simulink model "vof_control"  (R2022b)
settings: Solver=ode4  StartTime=0.0  StopTime=20  FixedStep=0.001  RelTol=1e-3
values from neighbouring files (symbols this model uses):
  Cm = [ones(1,r),zeros(1,r)]    [modal_control.m]
  Cv1 = ci*Cv    [modal_control.m]
  f = linspace(0, Fs/2, length(datos_filt)/2+1)    [FRF.m]    (also in FRFFrequencyResponseFunction.m; fft_Acelerometro.m = Fs*(0:(L/2))/L; fft_Mocap.m = Fs*(0:(L/2))/L; fftmocap.m = Fs*(0:(L/2))/L)
  fd = 8    [modal_control.m]
  gv = -2*w(i)*zetag/(bi*ci)    [modal_control.m]
  h = 1    [modal_control.m]
  k = 2*r    (= 10)    [modal_control.m]
  wn = sqrt(diag(eigenvalues))    [PironInternet.m]
undefined symbols (not defined in the file or in its folder): Am, Bm
settings Model: Creator=Jka  LastModifiedBy=raul
settings SolverCC: AlgebraicLoopSolver=TrustRegion
settings DebuggingCC: UnconnectedInputMsg=warning  UnconnectedOutputMsg=warning  UnconnectedLineMsg=warning  SFMachineParentedDataDiag=warning
settings ModelReferenceCC: EnableRefExpFcnMdlSchedulingChecks=on
settings RTWCC: DLArmComputeVersion=19.05

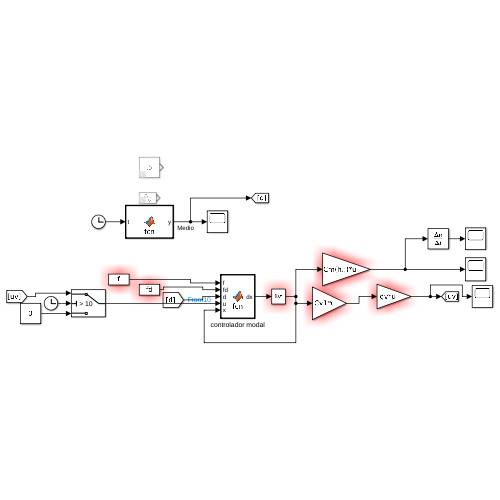
[thumbnail: Simulink's stored preview of the top-level diagram]
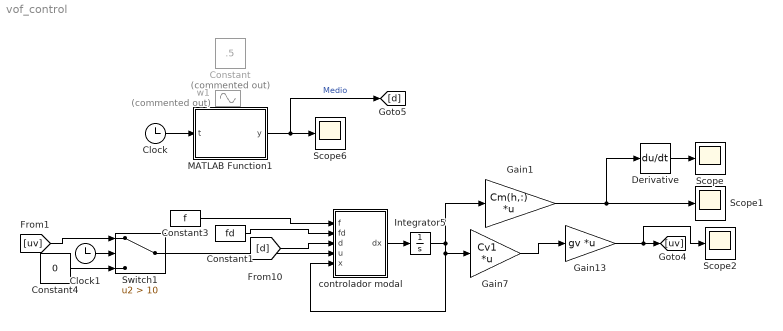
== system vof_control ==
  Clock : Clock
  Clock1 : Clock
  Constant : Constant  Commented=on  Value=.5
  Constant1 : Constant  Value=fd
  Constant3 : Constant  Value=f
  Constant4 : Constant  Value=0
  Derivative : Derivative
  Gain1 : Gain  Gain=Cm(h,:)  Multiplication=Matrix(K*u)
  Gain13 : Gain  Gain=gv  Multiplication=Matrix(K*u)
  Gain7 : Gain  Gain=Cv1  Multiplication=Matrix(K*u)
  Integrator5 : Integrator  InitialCondition=0*ones(k,1)
  MATLAB Function1 : MATLAB Function  TreatAsAtomicUnit=on
  Scope{,1..2,6} (4 alike) : Scope
  Switch1 : Switch  Criteria=u2 > Threshold  Threshold=10  SaturateOnIntegerOverflow=off  InputSameDT=off
  controlador modal : MATLAB Function  TreatAsAtomicUnit=on
  w1 : Sin  Commented=on  Frequency=wn(1)  Phase=pi/3  SampleTime=0
  wires:
  [d] -> controlador modal/3(d)
  controlador modal/1(dx) -> Integrator5/1
  Integrator5/1 -> controlador modal/5(x), Gain7/1, Gain1/1
  Gain13/1 -> Scope2/1, [uv]
  Constant3/1 -> controlador modal/1(f)
  Constant1/1 -> controlador modal/2(fd)
  Constant4/1 -> Switch1/3
  Clock1/1 -> Switch1/2
  [uv] -> Switch1/1
  Switch1/1 -> controlador modal/4(u)
  Gain1/1 -> Derivative/1, Scope1/1
  Gain7/1 -> Gain13/1
  Derivative/1 -> Scope/1
  MATLAB Function1/1(y) -> [d], Scope6/1  "Medio"
  Clock/1 -> MATLAB Function1/1(t)

== matlab function vof_control/MATLAB Function1 ==
  data: t input; y output
function y = fcn(t)


f=18.2185;
% f=120*(sin(t)+3.18);
% f=30;%frecuencia

%recordar que si para manipular f necesito t entonces y no debe tener t
% de lo contrario existirìa un t al cuadrado
y=1*(square(2*pi*f*t,50)+1);
end

== matlab function vof_control/controlador modal ==
  data: f input; fd input; d input; u input; x input; dx output; Am parameter; Bm parameter
function dx = fcn(f,fd,d,u,x,Am,Bm)
%#codegen

dx = Am*x+Bm(:,f)*u+Bm(:,fd)*d;
